simulink model "FINGERGame"  (Simulink 8.5)
settings: Solver=FixedStepDiscrete  StartTime=0.0  StopTime=inf  FixedStep=.001  RelTol=1e-3
PreLoadFcn:
  | settupFilter;
InitFcn:
  | settupFilter;
values from neighbouring files (symbols this model uses):
  x0low = (eye(size(Alow))-Alow)\Blow*0    [settupFilter.m]
undefined symbols (not defined in the file or in its folder): a_hp, Alow, b_hp, Blow, Clow, DiscIntNeverNeededParam, Dlow
libraries: slrtlib x8, simulink x5, xpcnilib x4
settings Model: Creator=Admin  LastModifiedBy=Juno  SimulationMode=external
settings SolverCC: EnableConcurrentExecution=on
settings DataIOCC: SignalLoggingSaveFormat=Dataset
settings OptimizationCC: BlockReduction=off  OptimizeBlockIOStorage=off  BufferReuse=off  GlobalBufferReuse=off  ExpressionFolding=off  LocalBlockOutputs=off
settings DebuggingCC: SolverPrmCheckMsg=warning  FcnCallInpInsideContextMsg=EnableAllAsError
settings HardwareCC: ProdIntDivRoundTo=Zero  ProdEndianess=LittleEndian  ProdLongLongMode=on  ProdHWDeviceType=Generic->32-bit x86 compatible
settings RTWCC: SystemTargetFile=slrt.tlc  TemplateMakefile=slrt_default_tmf  Description=Simulink Real-Time  RTWCompilerOptimization=on

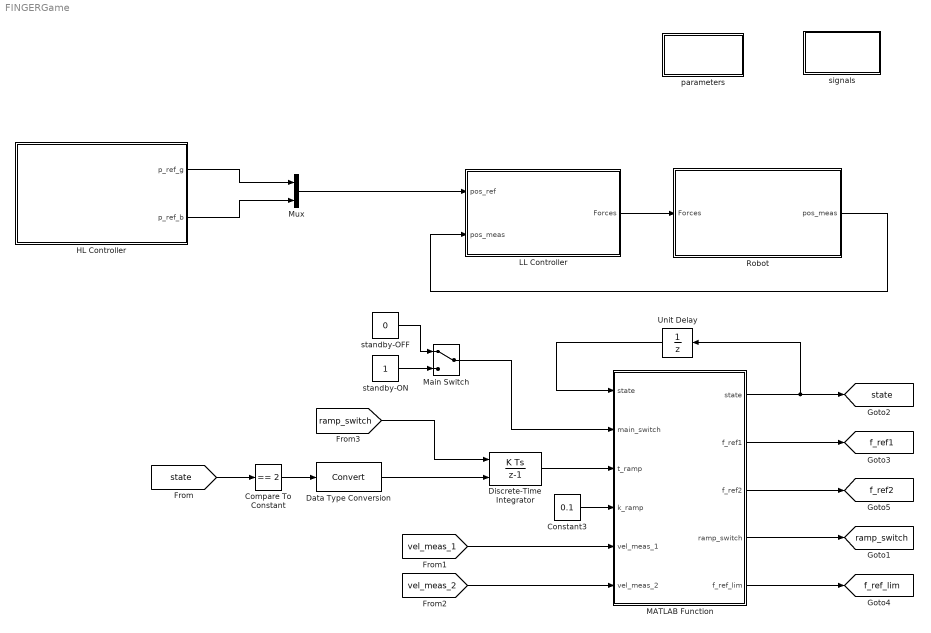
== system FINGERGame ==
  Compare To Constant : simulink/Logic and Bit Operations/Compare To Constant  relop===  const=2  OutDataTypeStr=boolean
  Constant3 : Constant  Value=0.1
  Data Type Conversion : DataTypeConversion
  Discrete-Time Integrator : DiscreteIntegrator  ExternalReset=either  InitialConditionSetting=State (most efficient)  SampleTime=-1  UpperSaturationLimit=0.9  LowerSaturationLimit=0  ICPrevOutput=DiscIntNeverNeededParam  ICPrevScaledInput=DiscIntNeverNeededParam
  HL Controller : Subsystem
  LL Controller : Subsystem
  MATLAB Function : MATLAB Function  TreatAsAtomicUnit=on
      settings: PermitHierarchicalResolution=ParametersOnly  MinAlgLoopOccurrences=on
  Main Switch : ManualSwitch
  Mux : Mux  Inputs=2
  Robot : Subsystem
  Unit Delay : UnitDelay  SampleTime=-1
  parameters : Subsystem
  signals : Subsystem
  standby-OFF : Constant  Value=0
  standby-ON : Constant
  tag scope: f_ref1=global, f_ref2=global, f_ref_lim=global, ramp_switch=global, state=global
  wires:
  LL Controller/1(Forces) -> Robot/1(Forces)
  HL Controller/1(p_ref_g) -> Mux/1
  HL Controller/2(p_ref_b) -> Mux/2
  Mux/1 -> LL Controller/1(pos_ref)
  Robot/1(pos_meas) -> LL Controller/2(pos_meas)
  MATLAB Function/1(state) -> Unit Delay/1, [state]
  Unit Delay/1 -> MATLAB Function/1("state ")
  standby-ON/1 -> Main Switch/2
  standby-OFF/1 -> Main Switch/1
  Main Switch/1 -> MATLAB Function/2(main_switch)
  MATLAB Function/2(f_ref1) -> [f_ref1]
  MATLAB Function/4(ramp_switch) -> [ramp_switch]
  Discrete-Time Integrator/1 -> MATLAB Function/3(t_ramp)
  Constant3/1 -> MATLAB Function/4(k_ramp)
  Compare To Constant/1 -> Data Type Conversion/1
  Data Type Conversion/1 -> Discrete-Time Integrator/2
  [state] -> Compare To Constant/1
  MATLAB Function/5(f_ref_lim) -> [f_ref_lim]
  [vel_meas_1] -> MATLAB Function/5(vel_meas_1)
  [vel_meas_2] -> MATLAB Function/6(vel_meas_2)
  [ramp_switch] -> Discrete-Time Integrator/1
  MATLAB Function/3(f_ref2) -> [f_ref2]

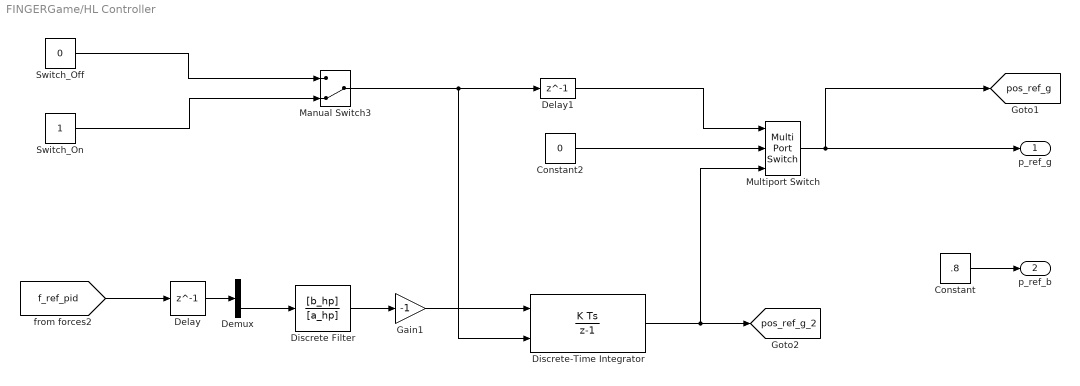
== system FINGERGame/HL Controller ==
  Constant : Constant  Value=.8
  Constant2 : Constant  Value=0
  Delay : Delay  DelayLength=1  InitialCondition=0
  Delay1 : Delay  DelayLength=1  InitialCondition=0
  Demux : Demux  Outputs=2
  Discrete Filter : DiscreteFilter  Numerator=[b_hp]  Denominator=[a_hp]
  Discrete-Time Integrator : DiscreteIntegrator  ExternalReset=either  InitialConditionSetting=State (most efficient)  SampleTime=-1  LimitOutput=on  UpperSaturationLimit=0.9  LowerSaturationLimit=0  ICPrevOutput=DiscIntNeverNeededParam  ICPrevScaledInput=DiscIntNeverNeededParam
  Gain1 : Gain  Gain=-1
  Manual Switch3 : ManualSwitch  CurrentSetting=0
  Multiport Switch : MultiPortSwitch  DataPortOrder=Specify indices  DataPortIndices={0,1}
  Switch_Off : Constant  Value=0
  Switch_On : Constant
  p_ref_g : Outport
  p_ref_b : Outport  Port=2
  tag scope: pos_ref_g=global, pos_ref_g_2=global
  wires:
  Discrete Filter/1 -> Gain1/1
  Constant/1 -> p_ref_b/1
  [f_ref_pid] -> Delay/1
  Gain1/1 -> Discrete-Time Integrator/1
  Multiport Switch/1 -> p_ref_g/1, [pos_ref_g]
  Manual Switch3/1 -> Discrete-Time Integrator/2, Delay1/1
  Switch_On/1 -> Manual Switch3/2
  Delay/1 -> Demux/1
  Demux/2 -> Discrete Filter/1
  Switch_Off/1 -> Manual Switch3/1
  Constant2/1 -> Multiport Switch/2
  Discrete-Time Integrator/1 -> Multiport Switch/3, [pos_ref_g_2]
  Delay1/1 -> Multiport Switch/1

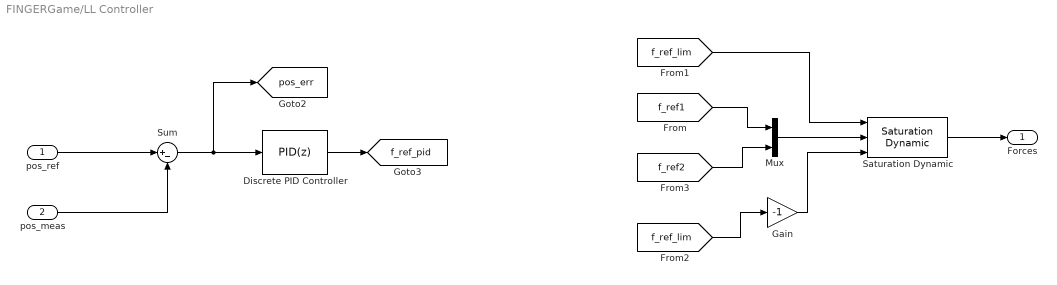
== system FINGERGame/LL Controller ==
  pos_ref : Inport
  pos_meas : Inport  Port=2
  Discrete PID Controller : simulink/Continuous/PID Controller  Controller=PID  TimeDomain=Discrete-time  SampleTime=-1  IntegratorMethod=Forward Euler  FilterMethod=Forward Euler  Form=Parallel  UseFilter=on  ControllerParametersSource=internal  P=10  I=0  D=0.7  N=100  InitialConditionSource=internal  InitialConditionForIntegrator=0  InitialConditionForFilter=0  ExternalReset=none  LimitOutput=off  UpperSaturationLimit=inf  LowerSaturationLimit=-inf  LinearizeAsGain=off  AntiWindupMode=none  Kb=1  TrackingMode=off  Kt=1  PParamMin=[]  PParamMax=[]  IParamMin=[]  IParamMax=[]  DParamMin=[]  DParamMax=[]  NParamMin=[]  NParamMax=[]  KbParamMin=[]  KbParamMax=[]  KtParamMin=[]  KtParamMax=[]  POutMin=[]  POutMax=[]  IOutMin=[]  IOutMax=[]  DOutMin=[]  DOutMax=[]  NOutMin=[]  NOutMax=[]  KbOutMin=[]  KbOutMax=[]  KtOutMin=[]  KtOutMax=[]  IntegratorOutMin=[]  IntegratorOutMax=[]  FilterOutMin=[]  FilterOutMax=[]  SumOutMin=[]  SumOutMax=[]  SumI1OutMin=[]  SumI1OutMax=[]  SumI2OutMin=[]  SumI2OutMax=[]  SumI3OutMin=[]  SumI3OutMax=[]  SumDOutMin=[]  SumDOutMax=[]  SaturationOutMin=[]  SaturationOutMax=[]  IntegratorContinuousStateAttributes=''  IntegratorStateMustResolveToSignalObject=off  IntegratorRTWStateStorageClass=Auto  FilterContinuousStateAttributes=''  FilterStateMustResolveToSignalObject=off  FilterRTWStateStorageClass=Auto  DifferentiatorICPrevScaledInput=0  DifferentiatorOutMin=[]  DifferentiatorOutMax=[]
  Gain : Gain  Gain=-1
  Mux : Mux  Inputs=2
  Saturation Dynamic : simulink/Discontinuities/Saturation Dynamic  OutMin=[]  OutMax=[]  OutDataTypeStr=Inherit: Same as second input  OutDataType=fixdt(1, 16)  OutScaling=2^-10  DoSatur=off
  Sum : Sum  Inputs=|+-
  Forces : Outport
  tag scope: f_ref_pid=global, pos_err=global
  wires:
  pos_meas/1 -> Sum/2
  Discrete PID Controller/1 -> [f_ref_pid]
  Sum/1 -> [pos_err], Discrete PID Controller/1
  pos_ref/1 -> Sum/1
  [f_ref_lim] -> Gain/1
  Saturation Dynamic/1 -> Forces/1
  [f_ref_lim] -> Saturation Dynamic/1
  Gain/1 -> Saturation Dynamic/3
  Mux/1 -> Saturation Dynamic/2
  [f_ref1] -> Mux/1
  [f_ref2] -> Mux/2

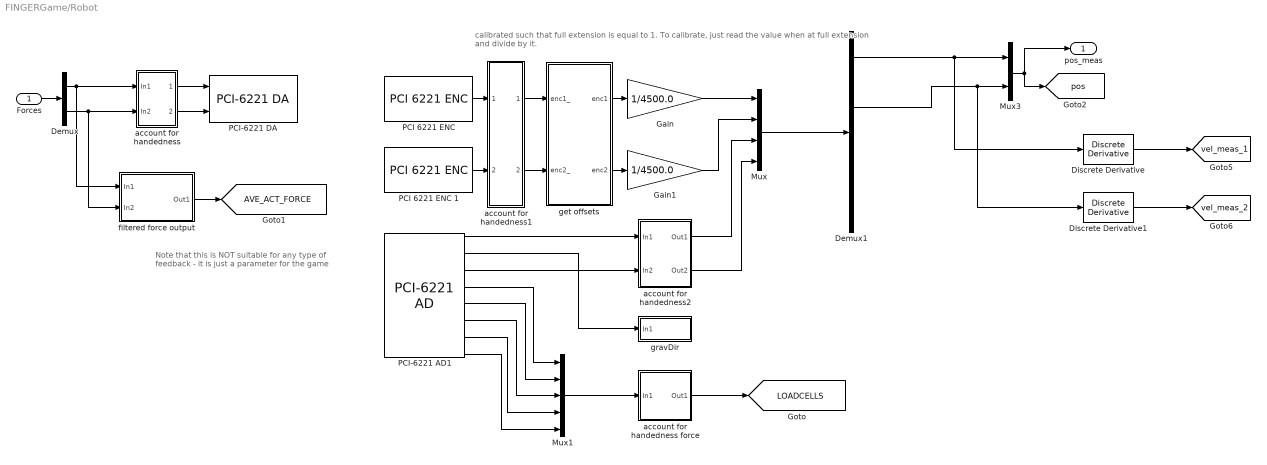
== system FINGERGame/Robot ==
  note: Note that this is NOT suitable for any type
      | of feedback - it is just a parameter for the game
  note: calibrated such that full extension is equal to 1. To calibrate, just read the value when at full extension and divide by it.
  Forces : Inport
  Demux : Demux  Outputs=2
  Demux1 : Demux
  Discrete Derivative : simulink/Discrete/Discrete Derivative  gainval=1.0  ICPrevScaledInput=0.0  OutMin=[]  OutMax=[]  OutDataType=fixdt(1, 16)  OutScaling=2^-10  DoSatur=off
  Discrete Derivative1 : simulink/Discrete/Discrete Derivative  gainval=1.0  ICPrevScaledInput=0.0  OutMin=[]  OutMax=[]  OutDataType=fixdt(1, 16)  OutScaling=2^-10  DoSatur=off
  Gain : Gain  Gain=1/4500.0
  Gain1 : Gain  Gain=1/4500.0
  Mux : Mux
  Mux1 : Mux  Inputs=5
  Mux3 : Mux  Inputs=2
  "PCI 6221 ENC " : xpcnilib/Incremental Encoder/PCI 6221 ENC   channel=0  countMode=Quadrature Mode x4  initCount=0  reload=off  indexPhase=A low B low  filter=Minimum pulse width 125 nanoseconds  sampleTime=0.001  slot=-1
  PCI 6221 ENC 1 : xpcnilib/Incremental Encoder/PCI 6221 ENC   channel=1  countMode=Quadrature Mode x4  initCount=0  reload=off  indexPhase=A low B low  filter=Minimum pulse width 125 nanoseconds  sampleTime=0.001  slot=-1
  PCI-6221 AD1 : xpcnilib/A//D/M Series/PCI-6221 AD  channel=[1 2 3 4 5 6 7 8]  range=[10]  coupling=[0]  scantime=5e-6  sampletime=0.001  slot=-1
  PCI-6221 DA : xpcnilib/D//A/M Series/PCI-6221 DA  channel=[1 2]  reset=[1]  initValue=[0]  sampletime=0.001  slot=-1
  account for handedness : Subsystem
  account for handedness force : Subsystem
  account for handedness1 : Subsystem
  account for handedness2 : Subsystem
  filtered force output : Subsystem
  get offsets : Subsystem
  gravDir : Subsystem
  pos_meas : Outport
  tag scope: AVE_ACT_FORCE=global, LOADCELLS=global, pos=global, vel_meas_1=global, vel_meas_2=global
  wires:
  Gain/1 -> Mux/1
  Forces/1 -> Demux/1
  Gain1/1 -> Mux/2
  get offsets/1(enc1) -> Gain/1
  get offsets/2(enc2) -> Gain1/1
  Demux/1 -> filtered force output/1(In1), account for handedness/1(In1)
  Demux/2 -> filtered force output/2(In2), account for handedness/2(In2)
  account for handedness/2(Out2) -> PCI-6221 DA/2
  account for handedness/1(Out1) -> PCI-6221 DA/1
  "PCI 6221 ENC "/1 -> account for handedness1/1(In1)
  account for handedness1/1(Out1) -> get offsets/1(enc1_)
  account for handedness1/2(Out2) -> get offsets/2(enc2_)
  PCI 6221 ENC 1/1 -> account for handedness1/2(In2)
  PCI-6221 AD1/1 -> account for handedness2/1(In1)
  PCI-6221 AD1/3 -> account for handedness2/2(In2)
  account for handedness2/1(Out1) -> Mux/3
  account for handedness2/2(Out2) -> Mux/4
  PCI-6221 AD1/4 -> Mux1/1
  PCI-6221 AD1/5 -> Mux1/2
  PCI-6221 AD1/6 -> Mux1/3
  PCI-6221 AD1/7 -> Mux1/4
  PCI-6221 AD1/8 -> Mux1/5
  Mux1/1 -> account for handedness force/1(In1)
  account for handedness force/1(Out1) -> [LOADCELLS]
  PCI-6221 AD1/2 -> gravDir/1(In1)
  filtered force output/1(Out1) -> [AVE_ACT_FORCE]
  Mux/1 -> Demux1/1
  Mux3/1 -> pos_meas/1, [pos]
  Demux1/1 -> Discrete Derivative/1, Mux3/1
  Demux1/2 -> Discrete Derivative1/1, Mux3/2
  Discrete Derivative/1 -> [vel_meas_1]
  Discrete Derivative1/1 -> [vel_meas_2]

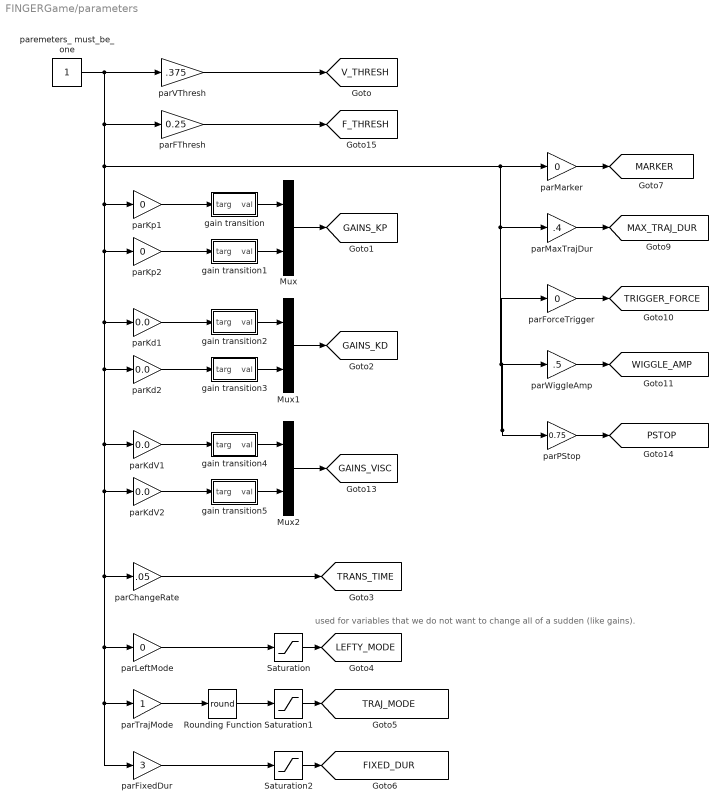
== system FINGERGame/parameters ==
  note: used for variables that we do not want to change all of a sudden (like gains).
  Mux : Mux  Inputs=2
  Mux1 : Mux  Inputs=2
  Mux2 : Mux  Inputs=2
  Rounding Function : Rounding  Operator=round
  Saturation : Saturate  UpperLimit=1  LowerLimit=0
  Saturation1 : Saturate  UpperLimit=4  LowerLimit=1
  Saturation2 : Saturate  UpperLimit=10  LowerLimit=.25
  gain transition : Subsystem
  gain transition1 : Subsystem
  gain transition2 : Subsystem
  gain transition3 : Subsystem
  gain transition4 : Subsystem
  gain transition5 : Subsystem
  parChangeRate : Gain  Gain=.05
  parFThresh : Gain  Gain=0.25
  parFixedDur : Gain  Gain=3
  parForceTrigger : Gain  Gain=0
  parKd1 : Gain  Gain=0.0
  parKd2 : Gain  Gain=0.0
  parKdV1 : Gain  Gain=0.0
  parKdV2 : Gain  Gain=0.0
  parKp1 : Gain  Gain=0
  parKp2 : Gain  Gain=0
  parLeftMode : Gain  Gain=0
  parMarker : Gain  Gain=0
  parMaxTrajDur : Gain  Gain=.4
  parPStop : Gain  Gain=0.75
  parTrajMode : Gain
  parVThresh : Gain  Gain=.375
  parWiggleAmp : Gain  Gain=.5
  paremeters_ must_be_one : Constant
  tag scope: FIXED_DUR=global, F_THRESH=global, GAINS_KD=global, GAINS_KP=global, GAINS_VISC=global, LEFTY_MODE=global, MARKER=global, MAX_TRAJ_DUR=global, PSTOP=global, TRAJ_MODE=global, TRANS_TIME=global, TRIGGER_FORCE=global, V_THRESH=global, WIGGLE_AMP=global
  wires:
  Mux/1 -> [GAINS_KP]
  Mux1/1 -> [GAINS_KD]
  Saturation/1 -> [LEFTY_MODE]
  gain transition/1(val) -> Mux/1
  gain transition1/1(val) -> Mux/2
  gain transition2/1(val) -> Mux1/1
  gain transition3/1(val) -> Mux1/2
  parVThresh/1 -> [V_THRESH]
  parKp1/1 -> gain transition/1(targ)
  parKp2/1 -> gain transition1/1(targ)
  parKd1/1 -> gain transition2/1(targ)
  parKd2/1 -> gain transition3/1(targ)
  parChangeRate/1 -> [TRANS_TIME]
  parLeftMode/1 -> Saturation/1
  Saturation1/1 -> [TRAJ_MODE]
  parTrajMode/1 -> Rounding Function/1
  Saturation2/1 -> [FIXED_DUR]
  parFixedDur/1 -> Saturation2/1
  Rounding Function/1 -> Saturation1/1
  parMarker/1 -> [MARKER]
  parMaxTrajDur/1 -> [MAX_TRAJ_DUR]
  parForceTrigger/1 -> [TRIGGER_FORCE]
  parWiggleAmp/1 -> [WIGGLE_AMP]
  Mux2/1 -> [GAINS_VISC]
  gain transition4/1(val) -> Mux2/1
  gain transition5/1(val) -> Mux2/2
  parKdV1/1 -> gain transition4/1(targ)
  parKdV2/1 -> gain transition5/1(targ)
  paremeters_ must_be_one/1 -> parVThresh/1, parFThresh/1, parKp1/1, parKp2/1, parKd1/1, parKd2/1, parKdV1/1, parKdV2/1, parChangeRate/1, parLeftMode/1, parFixedDur/1, parTrajMode/1, parPStop/1, parWiggleAmp/1, parForceTrigger/1, parMaxTrajDur/1, parMarker/1
  parPStop/1 -> [PSTOP]
  parFThresh/1 -> [F_THRESH]

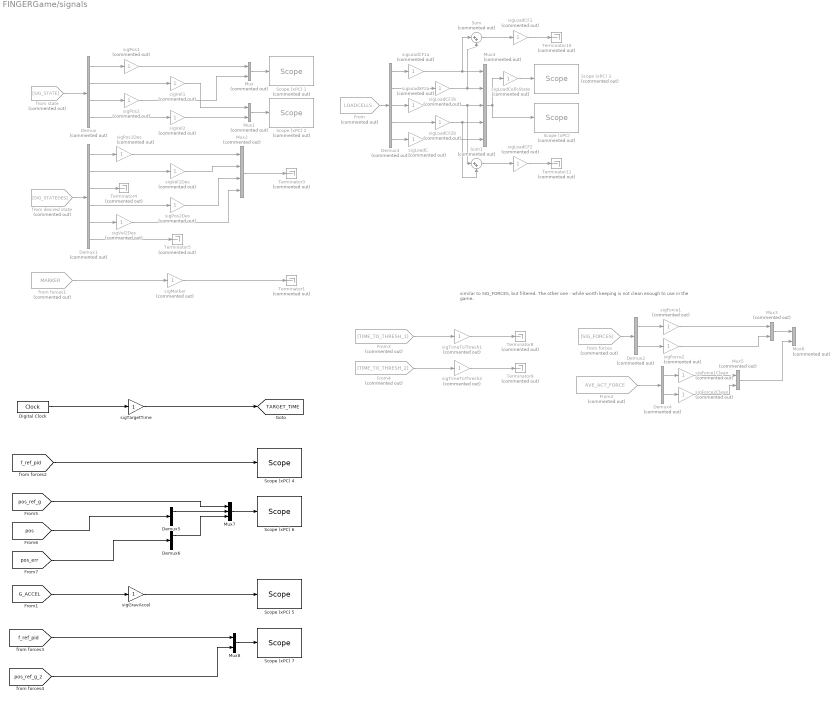
== system FINGERGame/signals ==
  note: similar to SIG_FORCES, but filtered. The other one - while worth keeping is not clean enough to use in the game.
  Demux : Demux  Commented=on
  Demux1 : Demux  Commented=on  Outputs=6
  Demux2 : Demux  Commented=on  Outputs=2
  Demux3 : Demux  Commented=on  Outputs=5
  Demux4 : Demux  Commented=on  Outputs=2
  Demux5 : Demux  Outputs=2
  Demux6 : Demux  Outputs=2
  Digital Clock : DigitalClock  SampleTime=.001
  From : From  Commented=on  GotoTag=LOADCELLS  TagVisibility=global
  From2 : From  Commented=on  GotoTag=AVE_ACT_FORCE  TagVisibility=global
  From3 : From  Commented=on  GotoTag=TIME_TO_THRESH_1
  From4 : From  Commented=on  GotoTag=TIME_TO_THRESH_2
  Mux{,1,3,5..6} (5 alike) : Mux  Commented=on  Inputs=2
  Mux2 : Mux  Commented=on
  Mux4 : Mux  Commented=on  Inputs=5
  Mux7 : Mux  Inputs=3
  Mux8 : Mux  Inputs=2
  "Scope (xPC) " : slrtlib/Displays and Logging/Scope   Commented=on  scopeno=5  scopetype=Target  autostart=on  viewmode=Graphical redraw  formatstr='%15.6f'  grid=on  ylimits=[-3,3]  nosamples=500  noprepostsamples=0  interleave=1  triggermode=FreeRun  triggersignal=1  trigsignalfromport=off  triggerlevel=0.0  triggerslope=Either  triggerscope=1  triggersample=0  filename=data.dat  mode=Lazy  writesize=512  autorestart=off  dynamicfilemode=off  maxwritefilesize=512*1024^2
  Scope (xPC) 1 : slrtlib/Displays and Logging/Scope   Commented=on  scopeno=1  scopetype=Target  autostart=on  viewmode=Graphical redraw  formatstr='%15.6f'  grid=on  ylimits=[0,1.1]  nosamples=500  noprepostsamples=0  interleave=1  triggermode=FreeRun  triggersignal=1  trigsignalfromport=off  triggerlevel=0.0  triggerslope=Either  triggerscope=1  triggersample=0  filename=data.dat  mode=Lazy  writesize=512  autorestart=off  dynamicfilemode=off  maxwritefilesize=512*1024^2
  Scope (xPC) 2 : slrtlib/Displays and Logging/Scope   Commented=on  scopeno=2  scopetype=Target  autostart=on  viewmode=Graphical redraw  formatstr='%15.6f'  grid=on  ylimits=[-10,10]  nosamples=500  noprepostsamples=0  interleave=1  triggermode=FreeRun  triggersignal=1  trigsignalfromport=off  triggerlevel=0.0  triggerslope=Either  triggerscope=1  triggersample=0  filename=data.dat  mode=Lazy  writesize=512  autorestart=off  dynamicfilemode=off  maxwritefilesize=512*1024^2
  Scope (xPC) 3 : slrtlib/Displays and Logging/Scope   Commented=on  scopeno=4  scopetype=File  autostart=on  viewmode=Graphical redraw  formatstr='%15.6f'  grid=on  ylimits=[0,0]  nosamples=5000  noprepostsamples=0  interleave=1  triggermode=FreeRun  triggersignal=1  trigsignalfromport=off  triggerlevel=0.0  triggerslope=Either  triggerscope=1  triggersample=0  filename=fLogData.dat  mode=Lazy  writesize=512  autorestart=off  dynamicfilemode=off  maxwritefilesize=512*1024^2
  Scope (xPC) 4 : slrtlib/Displays and Logging/Scope   scopeno=1  scopetype=Target  autostart=on  viewmode=Graphical rolling  formatstr='%15.6f'  grid=on  ylimits=[-1,1]  nosamples=2000  noprepostsamples=0  interleave=1  triggermode=FreeRun  triggersignal=1  trigsignalfromport=off  triggerlevel=0.0  triggerslope=Either  triggerscope=1  triggersample=0  filename=data.dat  mode=Lazy  writesize=512  autorestart=off  dynamicfilemode=off  maxwritefilesize=512*1024^2
  Scope (xPC) 5 : slrtlib/Displays and Logging/Scope   scopeno=2  scopetype=Target  autostart=on  viewmode=Graphical rolling  formatstr='%15.6f'  grid=on  ylimits=[-1,1]  nosamples=2000  noprepostsamples=0  interleave=1  triggermode=FreeRun  triggersignal=1  trigsignalfromport=off  triggerlevel=0.0  triggerslope=Either  triggerscope=1  triggersample=0  filename=data.dat  mode=Lazy  writesize=512  autorestart=off  dynamicfilemode=off  maxwritefilesize=512*1024^2
  Scope (xPC) 6 : slrtlib/Displays and Logging/Scope   scopeno=4  scopetype=Target  autostart=on  viewmode=Graphical rolling  formatstr='%15.6f'  grid=on  ylimits=[0,1]  nosamples=2000  noprepostsamples=0  interleave=1  triggermode=FreeRun  triggersignal=1  trigsignalfromport=off  triggerlevel=0.0  triggerslope=Either  triggerscope=1  triggersample=0  filename=data.dat  mode=Lazy  writesize=512  autorestart=off  dynamicfilemode=off  maxwritefilesize=512*1024^2
  Scope (xPC) 7 : slrtlib/Displays and Logging/Scope   scopeno=3  scopetype=Target  autostart=on  viewmode=Numerical  formatstr='%15.6f'  grid=on  ylimits=[.03,.1]  nosamples=10  noprepostsamples=0  interleave=1  triggermode=FreeRun  triggersignal=1  trigsignalfromport=off  triggerlevel=0.0  triggerslope=Either  triggerscope=1  triggersample=0  filename=data.dat  mode=Lazy  writesize=512  autorestart=off  dynamicfilemode=off  maxwritefilesize=512*1024^2
  Sum : Sum  Commented=on  Inputs=|++
  Sum1 : Sum  Commented=on  Inputs=|++
  Terminator{1,3..5,8..11} (8 alike) : Terminator  Commented=on
  from desired state : From  Commented=on  GotoTag=SIG_STATEDES
  from forces : From  Commented=on  GotoTag=SIG_FORCES  TagVisibility=global
  from forces1 : From  Commented=on  GotoTag=MARKER  TagVisibility=global
  from state : From  Commented=on  GotoTag=SIG_STATE  TagVisibility=global
  sigForce1 : Gain  Commented=on
  sigForce1Clean : Gain  Commented=on
  sigForce2 : Gain  Commented=on
  sigForce2Clean : Gain  Commented=on
  sigGravAccel : Gain
  sigLoadC : Gain  Commented=on
  sigLoadCF1 : Gain  Commented=on
  sigLoadCF1a : Gain  Commented=on
  sigLoadCF1b : Gain  Commented=on
  sigLoadCF2 : Gain  Commented=on
  sigLoadCF2a : Gain  Commented=on
  sigLoadCF2b : Gain  Commented=on
  sigLoadCellsState : Gain  Commented=on
  sigMarker : Gain  Commented=on
  sigPos1 : Gain  Commented=on
  sigPos1Des : Gain  Commented=on
  sigPos2 : Gain  Commented=on
  sigPos2Des : Gain  Commented=on
  sigTargetTime : Gain
  sigTimeToThresh1 : Gain  Commented=on
  sigTimeToThresh2 : Gain  Commented=on
  sigVel1 : Gain  Commented=on
  sigVel1Des : Gain  Commented=on
  sigVel2 : Gain  Commented=on
  sigVel2Des : Gain  Commented=on
  tag scope: TARGET_TIME=global
  wires:
  from state/1 -> Demux/1
  Demux/1 -> sigPos1/1
  Demux/2 -> sigVel1/1
  Demux/3 -> sigPos2/1
  Demux/4 -> sigVel2/1
  from desired state/1 -> Demux1/1
  Demux1/1 -> sigPos1Des/1
  Demux1/2 -> sigVel1Des/1
  Demux1/3 -> Terminator4/1
  Demux1/4 -> sigPos2Des/1
  Demux1/5 -> sigVel2Des/1
  Demux1/6 -> Terminator5/1
  Mux/1 -> Scope (xPC) 1/1
  Mux1/1 -> Scope (xPC) 2/1
  sigPos1/1 -> Mux/1
  sigPos2/1 -> Mux/2
  sigVel1/1 -> Mux1/1
  sigVel2/1 -> Mux1/2
  sigPos1Des/1 -> Mux2/1
  sigVel1Des/1 -> Mux2/2
  sigPos2Des/1 -> Mux2/3
  sigVel2Des/1 -> Mux2/4
  Mux2/1 -> Terminator3/1
  from forces/1 -> Demux2/1
  Demux2/1 -> sigForce1/1
  Demux2/2 -> sigForce2/1
  sigForce1/1 -> Mux3/1
  sigForce2/1 -> Mux3/2
  Digital Clock/1 -> sigTargetTime/1
  sigTargetTime/1 -> [TARGET_TIME]
  from forces1/1 -> sigMarker/1
  sigMarker/1 -> Terminator1/1
  From/1 -> Demux3/1
  Demux3/1 -> sigLoadCF1a/1
  Demux3/2 -> sigLoadCF1b/1
  Demux3/3 -> sigLoadCF2a/1
  Demux3/4 -> sigLoadCF2b/1
  Demux3/5 -> sigLoadC/1
  sigLoadCF1a/1 -> Sum/1, Mux4/1
  sigLoadCF1b/1 -> Sum/2, Mux4/2
  sigLoadCF2a/1 -> Sum1/1, Mux4/3
  sigLoadCF2b/1 -> Mux4/4, Sum1/2
  sigLoadC/1 -> Mux4/5
  Mux4/1 -> sigLoadCellsState/1, "Scope (xPC) "/1
  [G_ACCEL] -> sigGravAccel/1
  sigGravAccel/1 -> Scope (xPC) 5/1
  From2/1 -> Demux4/1
  Demux4/1 -> sigForce1Clean/1
  Demux4/2 -> sigForce2Clean/1
  sigForce1Clean/1 -> Mux5/1
  sigForce2Clean/1 -> Mux5/2
  sigTimeToThresh1/1 -> Terminator8/1
  From3/1 -> sigTimeToThresh1/1
  sigTimeToThresh2/1 -> Terminator9/1
  From4/1 -> sigTimeToThresh2/1
  sigLoadCellsState/1 -> Scope (xPC) 3/1
  Sum/1 -> sigLoadCF1/1
  Sum1/1 -> sigLoadCF2/1
  sigLoadCF1/1 -> Terminator10/1
  sigLoadCF2/1 -> Terminator11/1
  Mux3/1 -> Mux6/1
  Mux5/1 -> Mux6/2
  Mux7/1 -> Scope (xPC) 6/1
  [pos_ref_g] -> Mux7/1
  [f_ref_pid] -> Scope (xPC) 4/1
  [pos] -> Demux5/1
  Demux5/1 -> Mux7/2
  [pos_err] -> Demux6/1
  Demux6/1 -> Mux7/3
  Mux8/1 -> Scope (xPC) 7/1
  [f_ref_pid] -> Mux8/1
  [pos_ref_g_2] -> Mux8/2

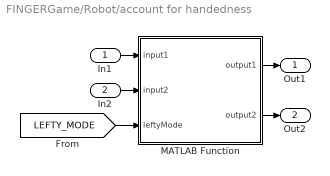
== system FINGERGame/Robot/account for handedness ==
  In1 : Inport
  In2 : Inport  Port=2
  MATLAB Function : MATLAB Function  TreatAsAtomicUnit=on
      settings: PermitHierarchicalResolution=ParametersOnly
  Out1 : Outport
  Out2 : Outport  Port=2
  wires:
  MATLAB Function/1(output1) -> Out1/1
  MATLAB Function/2(output2) -> Out2/1
  In1/1 -> MATLAB Function/1(input1)
  In2/1 -> MATLAB Function/2(input2)
  [LEFTY_MODE] -> MATLAB Function/3(leftyMode)

== system FINGERGame/Robot/account for handedness force ==
  In1 : Inport
  MATLAB Function : MATLAB Function  TreatAsAtomicUnit=on
      settings: PermitHierarchicalResolution=ParametersOnly
  Out1 : Outport
  wires:
  [LEFTY_MODE] -> MATLAB Function/2(leftyMode)
  MATLAB Function/1(output) -> Out1/1
  In1/1 -> MATLAB Function/1(inp1)

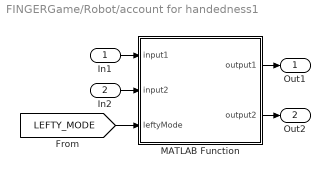
== system FINGERGame/Robot/account for handedness1 ==
  In1 : Inport
  In2 : Inport  Port=2
  MATLAB Function : MATLAB Function  TreatAsAtomicUnit=on
      settings: PermitHierarchicalResolution=ParametersOnly
  Out1 : Outport
  Out2 : Outport  Port=2
  wires:
  MATLAB Function/1(output1) -> Out1/1
  MATLAB Function/2(output2) -> Out2/1
  In1/1 -> MATLAB Function/1(input1)
  In2/1 -> MATLAB Function/2(input2)
  [LEFTY_MODE] -> MATLAB Function/3(leftyMode)

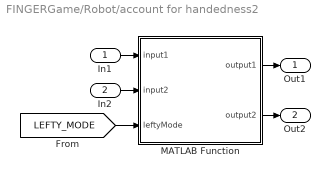
== system FINGERGame/Robot/account for handedness2 ==
  In1 : Inport
  In2 : Inport  Port=2
  MATLAB Function : MATLAB Function  TreatAsAtomicUnit=on
      settings: PermitHierarchicalResolution=ParametersOnly
  Out1 : Outport
  Out2 : Outport  Port=2
  wires:
  MATLAB Function/1(output1) -> Out1/1
  MATLAB Function/2(output2) -> Out2/1
  In1/1 -> MATLAB Function/1(input1)
  In2/1 -> MATLAB Function/2(input2)
  [LEFTY_MODE] -> MATLAB Function/3(leftyMode)

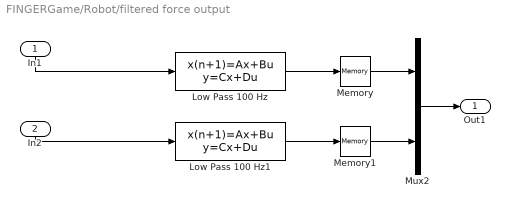
== system FINGERGame/Robot/filtered force output ==
  In1 : Inport
  In2 : Inport  Port=2
  Low Pass 100 Hz : DiscreteStateSpace  A=Alow  B=Blow  C=Clow  D=Dlow  X0=x0low  SampleTime=-1
  Low Pass 100 Hz1 : DiscreteStateSpace  A=Alow  B=Blow  C=Clow  D=Dlow  X0=x0low  SampleTime=-1
  Memory : Memory
  Memory1 : Memory
  Mux2 : Mux  Inputs=2
  Out1 : Outport
  wires:
  Low Pass 100 Hz1/1 -> Memory1/1
  Low Pass 100 Hz/1 -> Memory/1
  Mux2/1 -> Out1/1
  In1/1 -> Low Pass 100 Hz/1
  In2/1 -> Low Pass 100 Hz1/1
  Memory/1 -> Mux2/1
  Memory1/1 -> Mux2/2

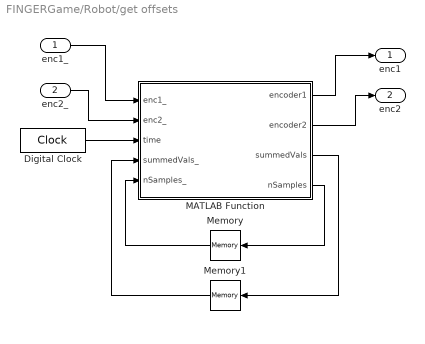
== system FINGERGame/Robot/get offsets ==
  enc1_ : Inport
  enc2_ : Inport  Port=2
  Digital Clock : DigitalClock  SampleTime=.001
  MATLAB Function : MATLAB Function  TreatAsAtomicUnit=on
      settings: PermitHierarchicalResolution=ParametersOnly
  Memory : Memory
  Memory1 : Memory  X0=[0,0]
  enc1 : Outport
  enc2 : Outport  Port=2
  wires:
  Memory/1 -> MATLAB Function/5(nSamples_)
  Memory1/1 -> MATLAB Function/4(summedVals_)
  MATLAB Function/3(summedVals) -> Memory1/1
  Digital Clock/1 -> MATLAB Function/3(time)
  MATLAB Function/1(encoder1) -> enc1/1
  MATLAB Function/2(encoder2) -> enc2/1
  enc2_/1 -> MATLAB Function/2(enc2_)
  enc1_/1 -> MATLAB Function/1(enc1_)
  MATLAB Function/4(nSamples) -> Memory/1

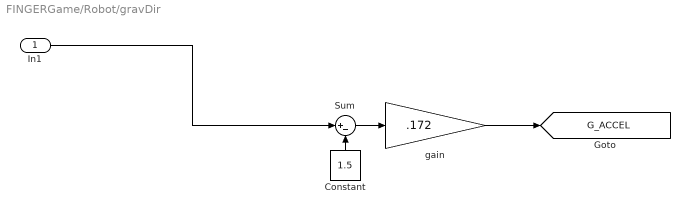
== system FINGERGame/Robot/gravDir ==
  In1 : Inport
  Constant : Constant  Value=1.5
  Sum : Sum  Inputs=|+-
  gain : Gain  Gain=.172
  tag scope: G_ACCEL=global
  wires:
  gain/1 -> [G_ACCEL]
  Sum/1 -> gain/1
  Constant/1 -> Sum/2
  In1/1 -> Sum/1

== system FINGERGame/parameters/gain transition ==
  targ : Inport
  Memory : Memory  X0=zeros(1,4)
  gainramp : MATLAB Function  TreatAsAtomicUnit=on
      settings: PermitHierarchicalResolution=ParametersOnly
  val : Outport
  wires:
  Memory/1 -> gainramp/3(state)
  gainramp/2(state1) -> Memory/1
  [TRANS_TIME] -> gainramp/1(tr)
  gainramp/1(val) -> val/1
  targ/1 -> gainramp/2(valD)

== system FINGERGame/parameters/gain transition1 ==
  targ : Inport
  Memory : Memory  X0=zeros(1,4)
  gainramp : MATLAB Function  TreatAsAtomicUnit=on
      settings: PermitHierarchicalResolution=ParametersOnly
  val : Outport
  wires:
  Memory/1 -> gainramp/3(state)
  gainramp/2(state1) -> Memory/1
  [TRANS_TIME] -> gainramp/1(tr)
  gainramp/1(val) -> val/1
  targ/1 -> gainramp/2(valD)

== system FINGERGame/parameters/gain transition2 ==
  targ : Inport
  Memory : Memory  X0=zeros(1,4)
  gainramp : MATLAB Function  TreatAsAtomicUnit=on
      settings: PermitHierarchicalResolution=ParametersOnly
  val : Outport
  wires:
  Memory/1 -> gainramp/3(state)
  gainramp/2(state1) -> Memory/1
  [TRANS_TIME] -> gainramp/1(tr)
  gainramp/1(val) -> val/1
  targ/1 -> gainramp/2(valD)

== system FINGERGame/parameters/gain transition3 ==
  targ : Inport
  Memory : Memory  X0=zeros(1,4)
  gainramp : MATLAB Function  TreatAsAtomicUnit=on
      settings: PermitHierarchicalResolution=ParametersOnly
  val : Outport
  wires:
  Memory/1 -> gainramp/3(state)
  gainramp/2(state1) -> Memory/1
  [TRANS_TIME] -> gainramp/1(tr)
  gainramp/1(val) -> val/1
  targ/1 -> gainramp/2(valD)

== system FINGERGame/parameters/gain transition4 ==
  targ : Inport
  Memory : Memory  X0=zeros(1,4)
  gainramp : MATLAB Function  TreatAsAtomicUnit=on
      settings: PermitHierarchicalResolution=ParametersOnly
  val : Outport
  wires:
  Memory/1 -> gainramp/3(state)
  gainramp/2(state1) -> Memory/1
  [TRANS_TIME] -> gainramp/1(tr)
  gainramp/1(val) -> val/1
  targ/1 -> gainramp/2(valD)

== system FINGERGame/parameters/gain transition5 ==
  targ : Inport
  Memory : Memory  X0=zeros(1,4)
  gainramp : MATLAB Function  TreatAsAtomicUnit=on
      settings: PermitHierarchicalResolution=ParametersOnly
  val : Outport
  wires:
  Memory/1 -> gainramp/3(state)
  gainramp/2(state1) -> Memory/1
  [TRANS_TIME] -> gainramp/1(tr)
  gainramp/1(val) -> val/1
  targ/1 -> gainramp/2(valD)

== matlab function MATLAB Function ==
  data: state input double; state output double; main_switch input double; f_ref1 output double; f_ref2 output double; ramp_switch output double; t_ramp input double; k_ramp input double; f_ref_lim output double; vel_meas_1 input double; vel_meas_2 input double
%% Create Finite State Machine for FINGER Robot 

function [state,f_ref1,f_ref2,ramp_switch,f_ref_lim] = StateMachine(state,main_switch,t_ramp,k_ramp,vel_meas_1,vel_meas_2)
%#codegen

ramp_switch = 0;


switch state
    
    case 1 %standby phase 
        f_ref1=0; % establish reference force
        f_ref2=0; % establish reference force 

        f_ref_lim=0; % establish limit for reference force 

        if main_switch==1  % If the main switch is on proceed to next state
            state=2;
        end
        
    case 2 %position zero  
        ramp_switch = 1; % Define value of ramp switch
        f_ref1=t_ramp*k_ramp; % Calculate reference force 
        f_ref2=t_ramp*k_ramp;
        f_ref_lim=5; % re-establish limit for reference force 

        if (vel_meas_1<0.001) && (vel_meas_2<0.001)
            state=3;
        end
        
    case 3 %Calibrate Encoder
        f_ref1=0;
        f_ref2=0;
        f_ref_lim =5; 
        ramp_switch = 0; 
   % case 4  %Operating Mode - Impaired Subjects
        % set the limits for the robot while in this mode here 
        % establish velocity limits here 
        % Implement the PID controllers here 
        % Imput Criteria to go from this mode to Emergency Shut Off Mode 
   % case 41 %Operating Mode - Healthy Subjects
        %set the limits for the robot while in this mode here 
        %establish velocity limits here 
        %Implement the PID controllers here 
        %Imput Criteria to go from this mode to Emergency Shut Off Mode
   % case 5 %Emergency Shut Off Mode
        % If error occurs while in either operating case shut off robot 
    %case 6 % Turn off Robot Mode
        % If movement ceases for x amount of time close program and shut
        % off robot
end
end

== matlab function Robot/get offsets/MATLAB Function ==
  data: enc1_ input double; encoder1 output double; enc2_ input double; time input double; summedVals_ input double; nSamples_ input double; encoder2 output double; summedVals output double; nSamples output double
%% remove the position offset that comes from using the encoders for
% feedback
%%
function [encoder1, encoder2, summedVals, nSamples] = getOffset(enc1_, enc2_, time, summedVals_, nSamples_)
%#codegen
summedVals = summedVals_;
if (time > 2) && (time < 3)
    summedVals(1) = summedVals_(1) + enc1_;
    summedVals(2) = summedVals_(2) + enc2_;
    nSamples = nSamples_ + 1;
    encoder1 = 0;
    encoder2 = 0;
elseif (time >=3)
    summedVals = summedVals_;
    nSamples = nSamples_;
    encoder1 = enc1_ - summedVals(1)/nSamples;
    encoder2 = enc2_ - summedVals(2)/nSamples;
else (time <= 2)
    summedVals = summedVals_;
    nSamples = nSamples_;
    encoder1 = 0;
    encoder2 = 0;
end

== matlab function Robot/account for handedness/MATLAB Function ==
  data: input1 input double; output1 output double; input2 input double; leftyMode input double; output2 output double
% encoder 1 and output 1 relate to the blue mechanism
% encoder 2, output 2 and accel 2 relate to the gold mechanism
% in right hand mode, we want the gold mechanism to control the index finger
% in left hand mode, we want the blue mechanism to control the index finger

% we wallways want the index finger to be finger 1

function [output1, output2] = fcn(input1, input2, leftyMode)
%#codegen
if leftyMode == 1
    output1 = input1;
    output2 = input2;
else
    output1 = input2;
    output2 = input1;
end

== matlab function Robot/account for handedness1/MATLAB Function ==
  data: input1 input double; output1 output double; input2 input double; leftyMode input double; output2 output double
% encoder 1 and output 1 relate to the blue mechanism
% encoder 2, output 2 and accel 2 relate to the gold mechanism
% in right hand mode, we want the gold mechanism to control the index finger
% in left hand mode, we want the blue mechanism to control the index finger

% we wallways want the index finger to be finger 1

function [output1, output2] = fcn(input1, input2, leftyMode)
%#codegen
if leftyMode == 1
    output1 = input1;
    output2 = input2;
else
    output1 = input2;
    output2 = input1;
end

== matlab function Robot/account for handedness2/MATLAB Function ==
  data: input1 input double; output1 output double; input2 input double; leftyMode input double; output2 output double
% encoder 1 and output 1 relate to the blue mechanism
% encoder 2, output 2 and accel 2 relate to the gold mechanism
% in right hand mode, we want the gold mechanism to control the index finger
% in left hand mode, we want the blue mechanism to control the index finger

% we wallways want the index finger to be finger 1

function [output1, output2] = fcn(input1, input2, leftyMode)
%#codegen
if leftyMode == 1
    output1 = input1;
    output2 = input2;
else
    output1 = input2;
    output2 = input1;
end

== matlab function parameters/gain transition/gainramp ==
  data: val output double; tr input double; valD input double; state1 output double; state input double
% state contains [valD_,val_,Ro_,t_]
function [val,state1] = fcn(tr,valD,state)
%#eml

% first we need to check if they have changed the desired Value
if ~ (valD == state(1))
    state(1) = valD;
    state(4) = 0;
    state(3) = state(1) - state(2);
end

t = state(4);
Ro = state(3);

if ((t <= tr) && (tr~=0))
    Rd = Ro - Ro*(10*(t)^3/(tr)^3 - 15*(t)^4/(tr)^4 + 6*(t)^5/(tr)^5);
else
    Rd = 0;
end

val = state(1) - Rd;
state(2) = val;
state(4) = t + .001;
state1 = state;

== matlab function parameters/gain transition1/gainramp ==
  data: val output double; tr input double; valD input double; state1 output double; state input double
% state contains [valD_,val_,Ro_,t_]
function [val,state1] = fcn(tr,valD,state)
%#eml

% first we need to check if they have changed the desired Value
if ~ (valD == state(1))
    state(1) = valD;
    state(4) = 0;
    state(3) = state(1) - state(2);
end

t = state(4);
Ro = state(3);

if ((t <= tr) && (tr~=0))
    Rd = Ro - Ro*(10*(t)^3/(tr)^3 - 15*(t)^4/(tr)^4 + 6*(t)^5/(tr)^5);
else
    Rd = 0;
end

val = state(1) - Rd;
state(2) = val;
state(4) = t + .001;
state1 = state;

== matlab function parameters/gain transition2/gainramp ==
  data: val output double; tr input double; valD input double; state1 output double; state input double
% state contains [valD_,val_,Ro_,t_]
function [val,state1] = fcn(tr,valD,state)
%#eml

% first we need to check if they have changed the desired Value
if ~ (valD == state(1))
    state(1) = valD;
    state(4) = 0;
    state(3) = state(1) - state(2);
end

t = state(4);
Ro = state(3);

if ((t <= tr) && (tr~=0))
    Rd = Ro - Ro*(10*(t)^3/(tr)^3 - 15*(t)^4/(tr)^4 + 6*(t)^5/(tr)^5);
else
    Rd = 0;
end

val = state(1) - Rd;
state(2) = val;
state(4) = t + .001;
state1 = state;

== matlab function parameters/gain transition3/gainramp ==
  data: val output double; tr input double; valD input double; state1 output double; state input double
% state contains [valD_,val_,Ro_,t_]
function [val,state1] = fcn(tr,valD,state)
%#eml

% first we need to check if they have changed the desired Value
if ~ (valD == state(1))
    state(1) = valD;
    state(4) = 0;
    state(3) = state(1) - state(2);
end

t = state(4);
Ro = state(3);

if ((t <= tr) && (tr~=0))
    Rd = Ro - Ro*(10*(t)^3/(tr)^3 - 15*(t)^4/(tr)^4 + 6*(t)^5/(tr)^5);
else
    Rd = 0;
end

val = state(1) - Rd;
state(2) = val;
state(4) = t + .001;
state1 = state;

== matlab function Robot/account for handedness force/MATLAB Function ==
  data: inp1 input double; output output double; leftyMode input double
% channel1 - gold tip
% channel2 - blue tip
% channel3 - gold base
% channel4 - blue base
% we wallways want the index finger to be finger 1

function output = fcn(inp1, leftyMode)
%#codegen

if leftyMode == 1
    output = [inp1(4); inp1(2); inp1(3); inp1(1); inp1(5)];
else
    output = [inp1(3); inp1(1); inp1(4); inp1(2); inp1(5)];
    %output = [inp1(3,1); inp1(4,2); inp1(5)];
end

== matlab function parameters/gain transition4/gainramp ==
  data: val output double; tr input double; valD input double; state1 output double; state input double
% state contains [valD_,val_,Ro_,t_]
function [val,state1] = fcn(tr,valD,state)
%#eml

% first we need to check if they have changed the desired Value
if ~ (valD == state(1))
    state(1) = valD;
    state(4) = 0;
    state(3) = state(1) - state(2);
end

t = state(4);
Ro = state(3);

if ((t <= tr) && (tr~=0))
    Rd = Ro - Ro*(10*(t)^3/(tr)^3 - 15*(t)^4/(tr)^4 + 6*(t)^5/(tr)^5);
else
    Rd = 0;
end

val = state(1) - Rd;
state(2) = val;
state(4) = t + .001;
state1 = state;

== matlab function parameters/gain transition5/gainramp ==
  data: val output double; tr input double; valD input double; state1 output double; state input double
% state contains [valD_,val_,Ro_,t_]
function [val,state1] = fcn(tr,valD,state)
%#eml

% first we need to check if they have changed the desired Value
if ~ (valD == state(1))
    state(1) = valD;
    state(4) = 0;
    state(3) = state(1) - state(2);
end

t = state(4);
Ro = state(3);

if ((t <= tr) && (tr~=0))
    Rd = Ro - Ro*(10*(t)^3/(tr)^3 - 15*(t)^4/(tr)^4 + 6*(t)^5/(tr)^5);
else
    Rd = 0;
end

val = state(1) - Rd;
state(2) = val;
state(4) = t + .001;
state1 = state;
